simulink model "acdc_nonstable"  (R2016a)
settings: Solver=FixedStepAuto  StartTime=0.0  StopTime=0.02  FixedStep=1e-7  RelTol=1e-3
libraries: powerlib x27, powerlib_meascontrol x3
settings Model: Creator=Lee  LastModifiedBy=Lee

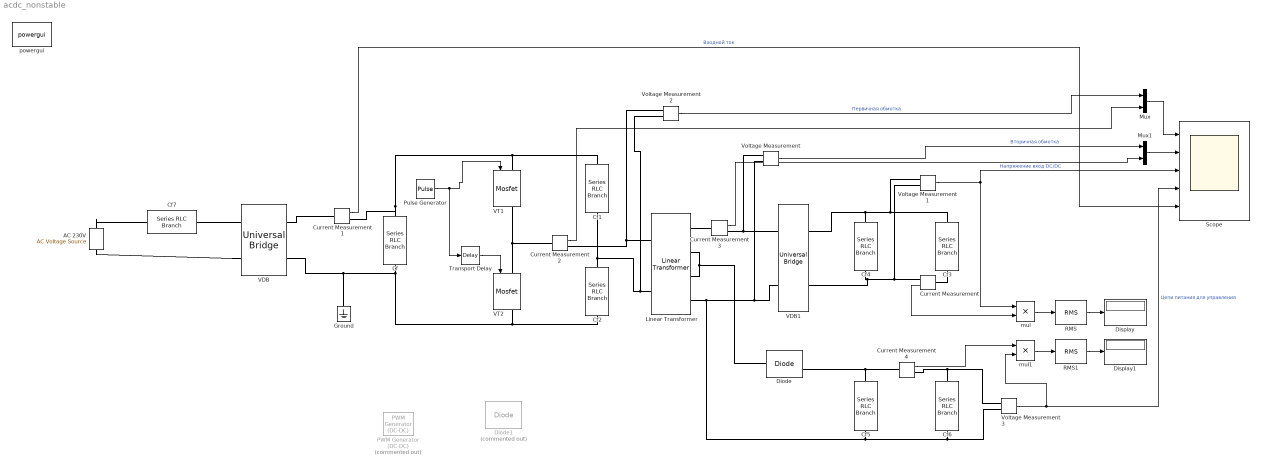
== system acdc_nonstable ==
  AC 230V : powerlib/Electrical Sources/AC Voltage Source  Amplitude=230*sqrt(2)  Phase=0  Frequency=60  SampleTime=0  Measurements=None  BusType=swing  Pref=10e3  Qref=0  Qmin=-inf  Qmax=+inf
  Cf : powerlib/Elements/Series RLC Branch  LConnTagsString=__new0  RConnTagsString=__new0  BranchType=C  Resistance=1  Inductance=1e-3  SetiL0=off  InitialCurrent=0  Capacitance=470e-6  Setx0=off  InitialVoltage=0  Measurements=None
  Cf1 : powerlib/Elements/Series RLC Branch  LConnTagsString=__new0  RConnTagsString=__new0  BranchType=C  Resistance=1  Inductance=1e-3  SetiL0=off  InitialCurrent=0  Capacitance=4.7e-6  Setx0=off  InitialVoltage=0  Measurements=None
  Cf2 : powerlib/Elements/Series RLC Branch  LConnTagsString=__new0  RConnTagsString=__new0  BranchType=C  Resistance=1  Inductance=1e-3  SetiL0=off  InitialCurrent=0  Capacitance=4.7e-6  Setx0=off  InitialVoltage=0  Measurements=None
  Cf3 : powerlib/Elements/Series RLC Branch  LConnTagsString=__new0  RConnTagsString=__new0  BranchType=R  Resistance=4.5  Inductance=1e-3  SetiL0=off  InitialCurrent=0  Capacitance=100e-6  Setx0=off  InitialVoltage=0  Measurements=None
  Cf4 : powerlib/Elements/Series RLC Branch  LConnTagsString=__new0  RConnTagsString=__new0  BranchType=C  Resistance=1  Inductance=1e-3  SetiL0=off  InitialCurrent=0  Capacitance=470e-6  Setx0=off  InitialVoltage=0  Measurements=None
  Cf5 : powerlib/Elements/Series RLC Branch  LConnTagsString=__new0  RConnTagsString=__new0  BranchType=C  Resistance=1  Inductance=1e-3  SetiL0=off  InitialCurrent=0  Capacitance=47e-6  Setx0=off  InitialVoltage=0  Measurements=None
  Cf6 : powerlib/Elements/Series RLC Branch  LConnTagsString=__new0  RConnTagsString=__new0  BranchType=R  Resistance=20  Inductance=1e-3  SetiL0=off  InitialCurrent=0  Capacitance=100e-6  Setx0=off  InitialVoltage=0  Measurements=None
  Cf7 : powerlib/Elements/Series RLC Branch  LConnTagsString=__new0  RConnTagsString=__new0  BranchType=R  Resistance=0.1  Inductance=1e-3  SetiL0=off  InitialCurrent=0  Capacitance=100e-6  Setx0=off  InitialVoltage=0  Measurements=None
  Current Measurement{,1..4} (5 alike) : powerlib/Measurements/Current Measurement  PhasorSimulation=off  OutputType=Complex  PSBequivalent=0
  Diode : powerlib/Power Electronics/Diode  Ron=0.005  Lon=0  Vf=0.6  IC=0  UseSnubber=off  Rs=500  Cs=250e-9  Measurements=on
  Diode1 : powerlib/Power Electronics/Diode  Commented=on  Ron=0.027  Lon=0  Vf=1.3  IC=0  UseSnubber=off  Rs=50000  Cs=250e-9  Measurements=on
  Display : Display
  Display1 : Display
  Ground : powerlib/Elements/Ground  LConnTagsString=a
  Linear Transformer : powerlib/Elements/Linear Transformer  UNITS=SI  NominalPower=[ 250e6 50 ]  winding1=[150 0.250 40e-6]  winding2=[37.5 0.05 10e-6]  ThreeWindings=on  winding3=[37.5 0.05 10e-6]  RmLm=[1.0805e+06 1e-3]  Measurements=None  DataType=on
  Mux : Mux  Inputs=2
  Mux1 : Mux  Inputs=2
  PWM Generator (DC-DC) : powerlib_meascontrol/Pulse & Signal Generators/PWM Generator (DC-DC)  Commented=on  Fsw=20000  Ts=0
  Pulse Generator : DiscretePulseGenerator  PulseType=Time based  Amplitude=10  Period=1/20000  PulseWidth=48
  RMS : powerlib_meascontrol/Measurements/RMS  TrueRMS=on  Freq=100  RMSInit=120  Ts=0
  RMS1 : powerlib_meascontrol/Measurements/RMS  TrueRMS=on  Freq=100  RMSInit=120  Ts=0
  Scope : Scope  NumInputPorts=5
  Transport Delay : TransportDelay  DelayTime=25e-6
  VDB : powerlib/Power Electronics/Universal Bridge  Arms=2  SnubberResistance=1e5  SnubberCapacitance=inf  Device=Diodes  Ron=5e-3  Lon=0  ForwardVoltages="[  0  0  ]"  ForwardVoltage=0.6  GTOparameters=[ 10e-6 , 20e-6 ]  IGBTparameters=[ 1e-6 , 2e-6 ]  Measurements=None  Measurements_2=None  converterType=Rectifier
  VDB1 : powerlib/Power Electronics/Universal Bridge  Arms=2  SnubberResistance=1e5  SnubberCapacitance=inf  Device=Diodes  Ron=5e-3  Lon=0  ForwardVoltages="[  0  0  ]"  ForwardVoltage=0.6  GTOparameters=[ 10e-6 , 20e-6 ]  IGBTparameters=[ 1e-6 , 2e-6 ]  Measurements=None  Measurements_2=None  converterType=Rectifier
  VT1 : powerlib/Power Electronics/Mosfet  Ron=0.6  Lon=0  Rd=0.01  Vfd=0.6  IC=0  Rs=1e5  Cs=inf  Measurements=on
  VT2 : powerlib/Power Electronics/Mosfet  Ron=0.6  Lon=0  Rd=0.01  Vfd=0.6  IC=0  Rs=1e5  Cs=inf  Measurements=on
  Voltage Measurement{,1..3} (4 alike) : powerlib/Measurements/Voltage Measurement  PhasorSimulation=off  OutputType=Complex  PSBequivalent=0
  mul : Product  Inputs=**
  mul1 : Product  Inputs=**
  powergui : powerlib/powergui  Priority=1  SimulationMode=Discrete  SolverType=Tustin/Backward Euler (TBE)  SampleTime=0.1e-6  frequency=60  SPID=off  DisableSnubberDevices=off  DisableRonSwitches=off  DisableVfSwitches=off  SwTol=0  DisplayEquations=off  Interpol=off  ExternalGateDelay=off  methode=off  Ts=10  FunctionMessages=off  echomessages=off  HookPort=off  EnableUseOfTLC=off  x0status=blocks  frequencyindice=0  Pbase=100e6  ErrMax=1e-4  Iterations=50  UnitsV=kV  UnitsW=MW  buscounter=0  RestoreLinks=warning  ResistiveCurrentMeasurement=off  Frange=[0:2:500]  Ylog=off  Xlog=on  ShowGrid=off  save=off  variable=ZData  structure=0  ZoomFFT=off  StartTime=0.0  cycles=1  DisplayStyle=1  fundamental=60  FreqAxis=off  MaxFrequency=1000  frequencyindicesteady=1  RmsSteady=1  display=off
  wires:
  Pulse Generator/1 -> Transport Delay/1, VT1/1
  Transport Delay/1 -> VT2/1
  Voltage Measurement/1 -> Mux1/1  "Вторичная обмотка"
  Voltage Measurement1/1 -> Scope/3, mul/1  "Напряжение вход DC/DC"
  Current Measurement/1 -> mul/2
  mul/1 -> RMS/1
  RMS/1 -> Display/1
  Voltage Measurement2/1 -> Mux/1  "Первичная обмотка"
  Voltage Measurement3/1 -> mul1/2, Scope/4  "Цепи питания для управления"
  Current Measurement1/1 -> Scope/5  "Входной ток"
  Current Measurement2/1 -> Mux/2
  Mux/1 -> Scope/1
  Mux1/1 -> Scope/2
  Current Measurement3/1 -> Mux1/2
  mul1/1 -> RMS1/1
  Current Measurement4/1 -> mul1/1
  RMS1/1 -> Display1/1
  connections:
  VDB/LConn2 -- AC 230V/LConn1
  Cf/RConn1 -- Ground/LConn1 -- VDB/RConn2 -- Cf2/RConn1 -- VT2/RConn1
  Cf/LConn1 -- Current Measurement1/RConn1 -- VT1/LConn1 -- Cf1/LConn1
  Cf2/LConn1 -- Voltage Measurement2/LConn2 -- Linear Transformer/LConn2 -- Cf1/RConn1
  Voltage Measurement/LConn1 -- Current Measurement3/RConn1 -- VDB1/LConn1
  Voltage Measurement1/LConn2 -- Current Measurement/RConn1 -- VDB1/RConn2 -- Cf4/RConn1
  Cf4/LConn1 -- VDB1/RConn1 -- Cf3/LConn1 -- Voltage Measurement1/LConn1
  Current Measurement/LConn1 -- Cf3/RConn1
  Linear Transformer/RConn2 -- Diode/LConn1 -- Linear Transformer/RConn3
  Cf5/LConn1 -- Diode/RConn1 -- Current Measurement4/LConn1
  Current Measurement1/LConn1 -- VDB/RConn1
  AC 230V/RConn1 -- Cf7/LConn1
  Cf7/RConn1 -- VDB/LConn1
  Linear Transformer/LConn1 -- Current Measurement2/RConn1 -- Voltage Measurement2/LConn1
  VT1/RConn1 -- Current Measurement2/LConn1 -- VT2/LConn1
  Linear Transformer/RConn1 -- Current Measurement3/LConn1
  Voltage Measurement/LConn2 -- VDB1/LConn2 -- Voltage Measurement3/LConn2 -- Cf6/RConn1 -- Cf5/RConn1 -- Linear Transformer/RConn4
  Voltage Measurement3/LConn1 -- Cf6/LConn1 -- Current Measurement4/RConn1
